simulink model "arducopter"  (R2021a)
settings: Solver=FixedStepAuto  StartTime=0.0  StopTime=sim.param.timeEnd  FixedStep=sim.param.dt  RelTol=1e-3
undefined symbols (not defined in the file or in its folder): DiscIntNeverNeededParam, sim
libraries: simulink x34, slident x4, vrlib x1
(part 4 of 8)

== system arducopter/Attitude Controller/input_euler_angle_roll_pitch_euler_rate_yaw()/update_ang_vel_target_from_att_error() ==
  note: The subsystems either use the square root controller or an easy proportional relation (kp*err) to calculate the target angular velocity
  note: AC_AttitudeControl::update_ang_vel_target_from_att_error()
      | Compute the angular velocity corrections in the body frame from the attitude error.
  attitudeError : Inport
  Calc angular velocity target pitch : Subsystem
  Calc angular velocity target roll : Subsystem
  Calc angular velocity target yaw : Subsystem
  Mux : Mux  Inputs=3
  Selector : Selector  InputPortWidth=3  IndexOptions=Index vector (dialog)  Indices=[1]  OutputSizes=1
  Selector1 : Selector  InputPortWidth=3  IndexOptions=Index vector (dialog)  Indices=[2]  OutputSizes=1
  Selector2 : Selector  InputPortWidth=3  IndexOptions=Index vector (dialog)  Indices=[3]  OutputSizes=1
  angVelBody : Outport
  wires:
  attitudeError/1 -> Selector2/1, Selector/1, Selector1/1
  Mux/1 -> angVelBody/1
  Selector/1 -> Calc angular velocity target roll/1(attitudeErrorRoll)
  Calc angular velocity target roll/1(angVelRoll) -> Mux/1
  Calc angular velocity target yaw/1(angVelYaw) -> Mux/3
  Calc angular velocity target pitch/1(angVelPitch) -> Mux/2
  Selector1/1 -> Calc angular velocity target pitch/1(attitudeErrorPitch)
  Selector2/1 -> Calc angular velocity target yaw/1(attitudeErrorYaw)

== system arducopter/Position Controller/P Position z/Scale Factor Z ==
  note: AP_AHRS::getControlScaleZ()
      | This subsystem calculates a scaling factor for the target of vertical motion quantities based on the EKF type that is being used.
      | Taken from AP_AHRS::getControlScaleZ() in AP_AHRS.cpp. Called in AC_PosControl::update_z_controller().
      | Flying with only DCM lower the gain of the controllers by 4x to cope with high lag.
  ekfType : Inport
  EKF used : Constant  OutDataTypeStr=single
  No EKF : Constant  Value=0.25  OutDataTypeStr=single
  Switch : Switch  Criteria=u2 > Threshold
  scale_z : Outport
  wires:
  ekfType/1 -> Switch/2
  EKF used/1 -> Switch/1
  No EKF/1 -> Switch/3
  Switch/1 -> scale_z/1

== system arducopter/Position Controller/P Position z/Set vertical speed & acceleration limit ==
  note: Calculation of vertical speed and acceleration limits
      | This subsystem corresponds to the function set_correction_speed_accel_z() , in AC_PosControl.cpp,
      | which is called in the ModeLoiter::init() function of mode_loiter.cpp.
      | The intention of this function is to calculate z position error limits, which corresponds to the vertical speed
      | and acceleration limits given by parameters, so that the speed and acceleration limits are still kept after
      | the square root controller was executed without explicitly enforce the limits to the quantities.
  outMin : Inport
  outMax : Inport  Port=2
  DoutMax : Inport  Port=3
  D2OutMax : Inport  Port=4
  kp : Inport  Port=5
  Abs : Abs
  Gain : Gain  Gain=-1
  Inverse Square Root Controller : Subsystem  TreatAsAtomicUnit=on
  Set error limits : MATLAB Function  TreatAsAtomicUnit=on
  errMin : Outport
  errMax : Outport  Port=2
  D1max : Outport  Port=3
  wires:
  Abs/1 -> Gain/1
  Gain/1 -> Set error limits/1(outMin)
  outMax/1 -> Set error limits/2(outMax)
  outMin/1 -> Abs/1
  DoutMax/1 -> Set error limits/3(DoutMax)
  Set error limits/1(errMin) -> errMin/1
  Set error limits/3(D1max) -> D1max/1
  Set error limits/2(errMax) -> errMax/1
  D2OutMax/1 -> Set error limits/4(D2OutMax)
  kp/1 -> Set error limits/5(kp)

== system arducopter/Position Controller/PID Acceleration z/Calc Derivative ==
  e : Inport
  ATC input time constant : Constant  Value=sim.param.dt
  Divide : Product  Inputs=*/
  Sum : Sum  Inputs=|+-
  Unit Delay : UnitDelay  SampleTime=-1  HasFrameUpgradeWarning=on
  derivative : Outport
  wires:
  e/1 -> Sum/1, Unit Delay/1
  Unit Delay/1 -> Sum/2
  Sum/1 -> Divide/1
  ATC input time constant/1 -> Divide/2
  Divide/1 -> derivative/1

== system arducopter/Position Controller/PID Acceleration z/I ==
  note: Integrator, see AC_PID.cpp, line 230
      | Initialization: set_integrator() in AC_PosControl::init_z_controller()
  e : Inport
  limitFlg : Inport  Port=2
  ki : Inport  Port=3
  i_max : Inport  Port=4
  Constant1 : Constant  Value=sim.param.dt
  Data Type Conversion1 : DataTypeConversion  OutDataTypeStr=single
  IC1 : InitialCondition  Value=sim.init.PIDA.I
  Integrator : MATLAB Function  TreatAsAtomicUnit=on
  Unit Delay1 : UnitDelay  InitialCondition=sim.init.PIDA.I  SampleTime=-1  HasFrameUpgradeWarning=on
  integrator : Outport
  wires:
  e/1 -> Integrator/1(error)
  Integrator/1(integrator_out) -> IC1/1
  [integrator_out] -> integrator/1
  Constant1/1 -> Data Type Conversion1/1
  limitFlg/1 -> Integrator/3(limit_flg)
  [integrator_out] -> Unit Delay1/1
  IC1/1 -> [integrator_out]
  Unit Delay1/1 -> Integrator/2(integrator)
  ki/1 -> Integrator/4(ki)
  i_max/1 -> Integrator/5(i_max)
  Data Type Conversion1/1 -> Integrator/6(dt)

== system arducopter/Position Controller/PID Acceleration z/RAT_FLTD ==
  note: Digital Filter:
      | $y_n = (1 - \alpha)y_{n-1} + x \cdot \alpha$
  note: Alpha Calculation:
      | $\alpha = \frac{\mathrm{d}t}{\mathrm{d}t + 2 \pi f_{\mathrm{Cutoff}}$
  note: See AC_PID.cpp, line 144.
  note: See AP_Math.cpp, line 393.
  u : Inport
  cutoff_freq : Inport  Port=2
  ATC input time constant : Constant  Value=sim.param.dt
  Add : Sum
  Calculate Alpha : Product  Inputs=*/
  Compare To Zero : simulink/Logic and Bit Operations/Compare To Zero  relop=<=  OutDataTypeStr=boolean
  Compare To Zero1 : simulink/Logic and Bit Operations/Compare To Zero  relop=<=  OutDataTypeStr=boolean
  Constant2 : Constant  OutDataTypeStr=single
  Constant3 : Constant  OutDataTypeStr=single
  Constant4 : Constant  OutDataTypeStr=single
  Data Type Conversion1 : DataTypeConversion  OutDataTypeStr=single
  Divide : Product  Inputs=*/
  Gain : Gain  Gain=2*pi
  IC : InitialCondition  Value=sim.init.PIDA.DerFilt
  Logical Operator : Logic  Operator=OR  AllPortsSameDT=off  OutDataTypeStr=boolean
  Product : Product
  Product1 : Product
  Subtract1 : Sum  Inputs=+-
  Sum : Sum  Inputs=++|  OutDataTypeStr=single
  Switch : Switch  Criteria=u2 > Threshold
  Unit Delay : UnitDelay  SampleTime=-1  HasFrameUpgradeWarning=on
  y : Outport
  wires:
  Product1/1 -> Sum/2
  Unit Delay/1 -> Product1/2
  Subtract1/1 -> Product1/1
  [alpha] -> Subtract1/2
  Constant2/1 -> Subtract1/1
  [alpha] -> Product/1
  Calculate Alpha/1 -> Switch/3
  Add/1 -> Calculate Alpha/2
  [dt] -> Add/1, Calculate Alpha/1
  Gain/1 -> Divide/2
  cutoff_freq/1 -> [cutoff_freq]
  u/1 -> Product/2
  Divide/1 -> Add/2
  Constant3/1 -> Divide/1
  Product/1 -> Sum/1
  Switch/1 -> [alpha]
  ATC input time constant/1 -> Data Type Conversion1/1
  [cutoff_freq] -> Gain/1
  [dt] -> Compare To Zero/1
  [cutoff_freq] -> Compare To Zero1/1
  Compare To Zero/1 -> Logical Operator/1
  Compare To Zero1/1 -> Logical Operator/2
  Logical Operator/1 -> Switch/2
  Constant4/1 -> Switch/1
  Sum/1 -> IC/1
  IC/1 -> Unit Delay/1, y/1
  Data Type Conversion1/1 -> [dt]

== system arducopter/Position Controller/PID Acceleration z/RAT_FLTE ==
  note: Digital Filter:
      | $y_n = (1 - \alpha)y_{n-1} + x \cdot \alpha$
  note: Alpha Calculation:
      | $\alpha = \frac{\mathrm{d}t}{\mathrm{d}t + 2 \pi f_{\mathrm{Cutoff}}$
  note: See AC_PID.cpp, line 144.
  note: See AP_Math.cpp, line 393.
  u : Inport
  cutoff_freq : Inport  Port=2
  ATC input time constant : Constant  Value=sim.param.dt
  Add : Sum
  Calculate Alpha : Product  Inputs=*/
  Compare To Zero : simulink/Logic and Bit Operations/Compare To Zero  relop=<=  OutDataTypeStr=boolean
  Compare To Zero1 : simulink/Logic and Bit Operations/Compare To Zero  relop=<=  OutDataTypeStr=boolean
  Constant2 : Constant  OutDataTypeStr=single
  Constant3 : Constant  OutDataTypeStr=single
  Constant4 : Constant  OutDataTypeStr=single
  Data Type Conversion1 : DataTypeConversion  OutDataTypeStr=single
  Divide : Product  Inputs=*/
  Gain : Gain  Gain=2*pi
  IC : InitialCondition  Value=sim.init.PIDA.ErrFilt
  Logical Operator : Logic  Operator=OR  AllPortsSameDT=off  OutDataTypeStr=boolean
  Product : Product
  Product1 : Product
  Subtract1 : Sum  Inputs=+-
  Sum : Sum  Inputs=++|  OutDataTypeStr=single
  Switch : Switch  Criteria=u2 > Threshold
  Unit Delay : UnitDelay  SampleTime=-1  HasFrameUpgradeWarning=on
  y : Outport
  wires:
  Product1/1 -> Sum/2
  Unit Delay/1 -> Product1/2
  Subtract1/1 -> Product1/1
  [alpha] -> Subtract1/2
  Constant2/1 -> Subtract1/1
  [alpha] -> Product/1
  Calculate Alpha/1 -> Switch/3
  Add/1 -> Calculate Alpha/2
  [dt] -> Add/1, Calculate Alpha/1
  Gain/1 -> Divide/2
  cutoff_freq/1 -> [cutoff_freq]
  u/1 -> Product/2
  Divide/1 -> Add/2
  Constant3/1 -> Divide/1
  Product/1 -> Sum/1
  Switch/1 -> [alpha]
  ATC input time constant/1 -> Data Type Conversion1/1
  [cutoff_freq] -> Gain/1
  [dt] -> Compare To Zero/1
  [cutoff_freq] -> Compare To Zero1/1
  Compare To Zero/1 -> Logical Operator/1
  Compare To Zero1/1 -> Logical Operator/2
  Logical Operator/1 -> Switch/2
  Constant4/1 -> Switch/1
  Sum/1 -> IC/1
  IC/1 -> Unit Delay/1, y/1
  Data Type Conversion1/1 -> [dt]

== system arducopter/Position Controller/PID Acceleration z/RAT_FLTT ==
  note: See AP_Math.cpp, line 393.
  note: See AC_PID.cpp, line 144.
  note: Alpha Calculation:
      | $\alpha = \frac{\mathrm{d}t}{\mathrm{d}t + 2 \pi f_{\mathrm{Cutoff}}$
  note: Digital Filter:
      | $y_n = (1 - \alpha)y_{n-1} + x \cdot \alpha$
  u : Inport
  cutoff_freq : Inport  Port=2
  ATC input time constant : Constant  Value=sim.param.dt
  Add : Sum
  Calculate Alpha : Product  Inputs=*/
  Compare To Zero : simulink/Logic and Bit Operations/Compare To Zero  relop=<=  OutDataTypeStr=boolean
  Compare To Zero1 : simulink/Logic and Bit Operations/Compare To Zero  relop=<=  OutDataTypeStr=boolean
  Constant2 : Constant  OutDataTypeStr=single
  Constant3 : Constant  OutDataTypeStr=single
  Constant4 : Constant  OutDataTypeStr=single
  Data Type Conversion1 : DataTypeConversion  OutDataTypeStr=single
  Divide : Product  Inputs=*/
  Gain : Gain  Gain=2*pi
  IC : InitialCondition  Value=sim.init.PIDA.TarFilt
  Logical Operator : Logic  Operator=OR  AllPortsSameDT=off  OutDataTypeStr=boolean
  Product : Product
  Product1 : Product
  Subtract1 : Sum  Inputs=+-
  Sum : Sum  Inputs=++|
  Switch : Switch  Criteria=u2 > Threshold
  Unit Delay : UnitDelay  SampleTime=-1  HasFrameUpgradeWarning=on
  y : Outport
  wires:
  Constant4/1 -> Switch/1
  Logical Operator/1 -> Switch/2
  Compare To Zero1/1 -> Logical Operator/2
  Compare To Zero/1 -> Logical Operator/1
  [cutoff_freq] -> Compare To Zero1/1
  [dt] -> Compare To Zero/1
  [cutoff_freq] -> Gain/1
  ATC input time constant/1 -> Data Type Conversion1/1
  Switch/1 -> [alpha]
  Product/1 -> Sum/1
  Constant3/1 -> Divide/1
  Divide/1 -> Add/2
  u/1 -> Product/2
  cutoff_freq/1 -> [cutoff_freq]
  Gain/1 -> Divide/2
  [dt] -> Calculate Alpha/1, Add/1
  Add/1 -> Calculate Alpha/2
  Calculate Alpha/1 -> Switch/3
  [alpha] -> Product/1
  Constant2/1 -> Subtract1/1
  [alpha] -> Subtract1/2
  Subtract1/1 -> Product1/1
  Product1/1 -> Sum/2
  Sum/1 -> IC/1
  Unit Delay/1 -> Product1/2
  IC/1 -> y/1, Unit Delay/1
  Data Type Conversion1/1 -> [dt]

== system arducopter/Position Controller/PID Acceleration z/Slew Limiter ==
  note: Data Store Memory Elements: Global variables of subsystem
  note: Slew Limiter
      |
      | Calculates the slew limit modifiert Dmod for the P and D part of the controller. The calculation of Dmod is taken from SlewLimiter::modifier() in SlewLimiter.cpp.
  p_out : Inport
  sr_max : Inport  Port=2
  sr_tau : Inport  Port=3
  sr_flt_f : Inport  Port=4
  clock : Inport  Port=5
  d_out : Inport  Port=6
  ATC sample time1 : Constant  Value=sim.param.dt
  Calculate Dmod : MATLAB Function  TreatAsAtomicUnit=on
  Constant7 : Constant  Value=sim.param.LOOP_RATE
  Data Store Memory : DataStoreMemory  DataStoreName=pos_event_stored  ReadBeforeWriteMsg=warning  WriteAfterWriteMsg=warning  WriteAfterReadMsg=warning  InitialValue=false  ShowAdditionalParam=off  OutDataTypeStr=boolean
  Data Store Memory1 : DataStoreMemory  DataStoreName=neg_event_stored  ReadBeforeWriteMsg=warning  WriteAfterWriteMsg=warning  WriteAfterReadMsg=warning  InitialValue=false  ShowAdditionalParam=off  OutDataTypeStr=boolean
  Data Store Memory10 : DataStoreMemory  DataStoreName=modifier_slew_rate  ReadBeforeWriteMsg=warning  WriteAfterWriteMsg=warning  WriteAfterReadMsg=warning  InitialValue=sim.init.PIDA.SROut  ShowAdditionalParam=off  OutDataTypeStr=single
  Data Store Memory11 : DataStoreMemory  DataStoreName=output_slew_rate  ReadBeforeWriteMsg=warning  WriteAfterWriteMsg=warning  WriteAfterReadMsg=warning  InitialValue=sim.init.PIDA.SROut  ShowAdditionalParam=off  OutDataTypeStr=single
  Data Store Memory2 : DataStoreMemory  DataStoreName=pos_event_idx  ReadBeforeWriteMsg=warning  WriteAfterWriteMsg=warning  WriteAfterReadMsg=warning  InitialValue=1  ShowAdditionalParam=off  OutDataTypeStr=int8
  Data Store Memory3 : DataStoreMemory  DataStoreName=neg_event_idx  ReadBeforeWriteMsg=warning  WriteAfterWriteMsg=warning  WriteAfterReadMsg=warning  InitialValue=1  ShowAdditionalParam=off  OutDataTypeStr=int8
  Data Store Memory4 : DataStoreMemory  DataStoreName=pos_event_ms  ReadBeforeWriteMsg=warning  WriteAfterWriteMsg=warning  WriteAfterReadMsg=warning  InitialValue=[0 0]  ShowAdditionalParam=off  OutDataTypeStr=uint32  Dimensions=2
  Data Store Memory5 : DataStoreMemory  DataStoreName=neg_event_ms  ReadBeforeWriteMsg=warning  WriteAfterWriteMsg=warning  WriteAfterReadMsg=warning  InitialValue=[0 0]  ShowAdditionalParam=off  OutDataTypeStr=uint32  Dimensions=2
  Data Store Memory6 : DataStoreMemory  DataStoreName=max_pos_slew_rate  ReadBeforeWriteMsg=warning  WriteAfterWriteMsg=warning  WriteAfterReadMsg=warning  ShowAdditionalParam=off  OutDataTypeStr=single
  Data Store Memory7 : DataStoreMemory  DataStoreName=max_pos_slew_event_ms  ReadBeforeWriteMsg=warning  WriteAfterWriteMsg=warning  WriteAfterReadMsg=warning  ShowAdditionalParam=off  OutDataTypeStr=uint32
  Data Store Memory8 : DataStoreMemory  DataStoreName=max_neg_slew_rate  ReadBeforeWriteMsg=warning  WriteAfterWriteMsg=warning  WriteAfterReadMsg=warning  ShowAdditionalParam=off  OutDataTypeStr=single
  Data Store Memory9 : DataStoreMemory  DataStoreName=max_neg_slew_event_ms  ReadBeforeWriteMsg=warning  WriteAfterWriteMsg=warning  WriteAfterReadMsg=warning  ShowAdditionalParam=off  OutDataTypeStr=uint32
  Data Store Read : DataStoreRead  DataStoreName=modifier_slew_rate  DataStoreElements=modifier_slew_rate  IndexOptions=Index vector (dialog)  Indices=1  OutputSizes=1
  Data Store Read1 : DataStoreRead  DataStoreName=output_slew_rate  DataStoreElements=output_slew_rate  IndexOptions=Index vector (dialog)  Indices=1  OutputSizes=1
  Data Type Conversion1 : DataTypeConversion  OutDataTypeStr=single
  IC : InitialCondition  Value=2*sim.init.PIDA.SROut
  Lowpass Filter : MATLAB Function  TreatAsAtomicUnit=on
  Subsystem : Subsystem
  Terminator : Terminator
  Terminator1 : Terminator
  Unit Delay1 : UnitDelay  SampleTime=-1  HasFrameUpgradeWarning=on
  Dmod : Outport
  wires:
  Constant7/1 -> Lowpass Filter/3(loop_rate)
  sr_flt_f/1 -> Lowpass Filter/2(cutoff_freq)
  Lowpass Filter/1(out) -> IC/1  "zAccSrFilt"
  Unit Delay1/1 -> Lowpass Filter/4(out_last)
  Calculate Dmod/1(Dmod) -> Dmod/1  "zAccDmod"
  sr_max/1 -> Calculate Dmod/2(sr_max)
  sr_tau/1 -> Calculate Dmod/3(sr_tau)
  ATC sample time1/1 -> Data Type Conversion1/1
  Data Store Read/1 -> Terminator/1  "zAccSrMod"
  Data Store Read1/1 -> Terminator1/1  "zAccSrOut"
  p_out/1 -> Subsystem/1(p_out)
  d_out/1 -> Subsystem/2(d_out)
  Subsystem/1(sr_raw) -> Lowpass Filter/1(in)  "zAccSrRaw"
  Data Type Conversion1/1 -> Calculate Dmod/4(dt)
  IC/1 -> Unit Delay1/1, Calculate Dmod/1(slew_rate)
  clock/1 -> Calculate Dmod/5(time)

== system arducopter/Position Controller/PID Acceleration z/i_max check ==
  note: Ensure imax is always large enough to overpower hover throttle
      | Check for sufficient high imax is taken from AC_PosControl.cpp, line 984-986.
  thrHover : Inport
  i_max_ : Inport  Port=2
  Gain : Gain  Gain=1000
  Relational Operator : RelationalOperator  Operator=>  OutDataTypeStr=boolean  RndMeth=Simplest
  Switch : Switch  Criteria=u2 > Threshold
  i_max : Outport
  wires:
  thrHover/1 -> Gain/1
  Gain/1 -> Switch/1, Relational Operator/1
  i_max_/1 -> Switch/3, Relational Operator/2
  Relational Operator/1 -> Switch/2
  Switch/1 -> i_max/1

== system arducopter/Position Controller/PID Velocity z/Calc Derivative ==
  e : Inport
  ATC input time constant : Constant  Value=sim.param.dt
  Divide : Product  Inputs=*/
  Sum : Sum  Inputs=|+-
  Unit Delay : UnitDelay  SampleTime=-1  HasFrameUpgradeWarning=on
  derivative : Outport
  wires:
  e/1 -> Sum/1, Unit Delay/1
  Unit Delay/1 -> Sum/2
  Sum/1 -> Divide/1
  ATC input time constant/1 -> Divide/2
  Divide/1 -> derivative/1

== system arducopter/Position Controller/PID Velocity z/I ==
  note: Integrator, see AC_PID_Basic::update_i()
      | Initialization: integrator=0 (see AC_PosControl::init_z())
  e : Inport
  limitNeg : Inport  Port=2
  limitPos : Inport  Port=3
  ki : Inport  Port=4
  i_max : Inport  Port=5
  Constant1 : Constant  Value=sim.param.dt
  Data Type Conversion1 : DataTypeConversion  OutDataTypeStr=single
  IC1 : InitialCondition  Value=0
  Integrator : MATLAB Function  TreatAsAtomicUnit=on
  Unit Delay1 : UnitDelay  InitialCondition=single(0)  SampleTime=-1  HasFrameUpgradeWarning=on
  integrator : Outport
  wires:
  e/1 -> Integrator/1(error)
  Integrator/1(integrator_out) -> IC1/1
  [integrator_out] -> integrator/1
  Constant1/1 -> Data Type Conversion1/1
  limitNeg/1 -> Integrator/3(limitNeg)
  [integrator_out] -> Unit Delay1/1
  IC1/1 -> [integrator_out]
  Unit Delay1/1 -> Integrator/2(integrator)
  ki/1 -> Integrator/5(ki)
  i_max/1 -> Integrator/6(i_max)
  Data Type Conversion1/1 -> Integrator/7(dt)
  limitPos/1 -> Integrator/4(limitPos)

== system arducopter/Position Controller/PID Velocity z/RAT_FLTD ==
  note: Digital Filter:
      | $y_n = (1 - \alpha)y_{n-1} + x \cdot \alpha$
  note: Alpha Calculation:
      | $\alpha = \frac{\mathrm{d}t}{\mathrm{d}t + 2 \pi f_{\mathrm{Cutoff}}$
  note: See AC_PID.cpp, update_all()
  note: See AP_Math.cpp, calc_lowpass_alpha_dt()
  u : Inport
  cutoff_freq : Inport  Port=2
  ATC input time constant : Constant  Value=sim.param.dt
  Add : Sum
  Calculate Alpha : Product  Inputs=*/
  Compare To Zero : simulink/Logic and Bit Operations/Compare To Zero  relop=<=  OutDataTypeStr=boolean
  Compare To Zero1 : simulink/Logic and Bit Operations/Compare To Zero  relop=<=  OutDataTypeStr=boolean
  Constant2 : Constant  OutDataTypeStr=single
  Constant3 : Constant  OutDataTypeStr=single
  Constant4 : Constant  OutDataTypeStr=single
  Data Type Conversion1 : DataTypeConversion  OutDataTypeStr=single
  Divide : Product  Inputs=*/
  Gain : Gain  Gain=2*pi
  IC : InitialCondition  Value=0
  Logical Operator : Logic  Operator=OR  AllPortsSameDT=off  OutDataTypeStr=boolean
  Product : Product
  Product1 : Product
  Subtract1 : Sum  Inputs=+-
  Sum : Sum  Inputs=++|  OutDataTypeStr=single
  Switch : Switch  Criteria=u2 > Threshold
  Unit Delay : UnitDelay  SampleTime=-1  HasFrameUpgradeWarning=on
  y : Outport
  wires:
  Product1/1 -> Sum/2
  Unit Delay/1 -> Product1/2
  Subtract1/1 -> Product1/1
  [alpha] -> Subtract1/2
  Constant2/1 -> Subtract1/1
  [alpha] -> Product/1
  Calculate Alpha/1 -> Switch/3
  Add/1 -> Calculate Alpha/2
  [dt] -> Add/1, Calculate Alpha/1
  Gain/1 -> Divide/2
  cutoff_freq/1 -> [cutoff_freq]
  u/1 -> Product/2
  Divide/1 -> Add/2
  Constant3/1 -> Divide/1
  Product/1 -> Sum/1
  Switch/1 -> [alpha]
  ATC input time constant/1 -> Data Type Conversion1/1
  [cutoff_freq] -> Gain/1
  [dt] -> Compare To Zero/1
  [cutoff_freq] -> Compare To Zero1/1
  Compare To Zero/1 -> Logical Operator/1
  Compare To Zero1/1 -> Logical Operator/2
  Logical Operator/1 -> Switch/2
  Constant4/1 -> Switch/1
  Sum/1 -> IC/1
  IC/1 -> Unit Delay/1, y/1
  Data Type Conversion1/1 -> [dt]

== system arducopter/Position Controller/PID Velocity z/RAT_FLTE ==
  note: Digital Filter:
      | $y_n = (1 - \alpha)y_{n-1} + x \cdot \alpha$
  note: Alpha Calculation:
      | $\alpha = \frac{\mathrm{d}t}{\mathrm{d}t + 2 \pi f_{\mathrm{Cutoff}}$
  note: See AC_PID.cpp, update_all()
  note: See AP_Math.cpp, calc_lowpass_alpha_dt()
  u : Inport
  cutoff_freq : Inport  Port=2
  ATC input time constant : Constant  Value=sim.param.dt
  Add : Sum
  Calculate Alpha : Product  Inputs=*/
  Compare To Zero : simulink/Logic and Bit Operations/Compare To Zero  relop=<=  OutDataTypeStr=boolean
  Compare To Zero1 : simulink/Logic and Bit Operations/Compare To Zero  relop=<=  OutDataTypeStr=boolean
  Constant2 : Constant  OutDataTypeStr=single
  Constant3 : Constant  OutDataTypeStr=single
  Constant4 : Constant  OutDataTypeStr=single
  Data Type Conversion1 : DataTypeConversion  OutDataTypeStr=single
  Divide : Product  Inputs=*/
  Gain : Gain  Gain=2*pi
  IC : InitialCondition  Value=0
  Logical Operator : Logic  Operator=OR  AllPortsSameDT=off  OutDataTypeStr=boolean
  Product : Product
  Product1 : Product
  Subtract1 : Sum  Inputs=+-
  Sum : Sum  Inputs=++|  OutDataTypeStr=single
  Switch : Switch  Criteria=u2 > Threshold
  Unit Delay : UnitDelay  SampleTime=-1  HasFrameUpgradeWarning=on
  y : Outport
  wires:
  Product1/1 -> Sum/2
  Unit Delay/1 -> Product1/2
  Subtract1/1 -> Product1/1
  [alpha] -> Subtract1/2
  Constant2/1 -> Subtract1/1
  [alpha] -> Product/1
  Calculate Alpha/1 -> Switch/3
  Add/1 -> Calculate Alpha/2
  [dt] -> Add/1, Calculate Alpha/1
  Gain/1 -> Divide/2
  cutoff_freq/1 -> [cutoff_freq]
  u/1 -> Product/2
  Divide/1 -> Add/2
  Constant3/1 -> Divide/1
  Product/1 -> Sum/1
  Switch/1 -> [alpha]
  ATC input time constant/1 -> Data Type Conversion1/1
  [cutoff_freq] -> Gain/1
  [dt] -> Compare To Zero/1
  [cutoff_freq] -> Compare To Zero1/1
  Compare To Zero/1 -> Logical Operator/1
  Compare To Zero1/1 -> Logical Operator/2
  Logical Operator/1 -> Switch/2
  Constant4/1 -> Switch/1
  Sum/1 -> IC/1
  IC/1 -> Unit Delay/1, y/1
  Data Type Conversion1/1 -> [dt]

== system arducopter/Position Controller/PID Velocity z/Scale Factor Z ==
  note: AP_AHRS::getControlScaleZ()
      | This subsystem calculates a scaling factor for the target of vertical motion quantities based on the EKF type that is being used.
      | Taken from AP_AHRS::getControlScaleZ() in AP_AHRS.cpp. Called in AC_PosControl::update_z_controller().
      | Flying with only DCM lower the gain of the controllers by 4x to cope with high lag.
  ekfType : Inport
  EKF used : Constant  OutDataTypeStr=single
  No EKF : Constant  Value=0.25  OutDataTypeStr=single
  Switch : Switch  Criteria=u2 > Threshold
  scale_z : Outport
  wires:
  ekfType/1 -> Switch/2
  EKF used/1 -> Switch/1
  No EKF/1 -> Switch/3
  Switch/1 -> scale_z/1

== system arducopter/Position Controller/calc des climb rate/contrain climb rate ==
  note: Based on get_pilot_speed_dn()
      | Use maximum up-speed if down-speed limit is 0
  in : Inport
  Abs : Abs
  Abs1 : Abs
  Constant1 : Constant  Value=sim.param.PSCD.VEL_MAX_DN
  Constant2 : Constant  Value=sim.param.PSCD.VEL_MAX_UP
  Constant3 : Constant  Value=sim.param.PSCD.VEL_MAX_UP
  Gain : Gain  Gain=-1
  Saturation Dynamic : simulink/Discontinuities/Saturation Dynamic  OutMin=[]  OutMax=[]  OutDataTypeStr=Inherit: Same as second input  OutDataType=fixdt(1, 16)  OutScaling=2^-10  DoSatur=off
  Switch : Switch  Criteria=u2 > Threshold
  out : Outport
  wires:
  Constant1/1 -> Abs/1, Switch/2
  Constant2/1 -> Abs1/1
  Abs/1 -> Switch/1
  Abs1/1 -> Switch/3
  Saturation Dynamic/1 -> out/1
  Switch/1 -> Gain/1
  Gain/1 -> Saturation Dynamic/3
  in/1 -> Saturation Dynamic/2
  Constant3/1 -> Saturation Dynamic/1

== system arducopter/Position Controller/set_pos_target_z_from_climb_rate()/input_vel_accel_z ==
  note: input_vel_accel_z()
      | This subsystem takes the current target position (posTarIn) and desired velocity and acceleration (velDesTar and accDesTar).
      | First, it updates the target position and desired velocity based on the current desired acceleration (accDesIn) (1).
      | Secondly, it calculates the required jerk limited adjustment to the acceleration for the next time dt (accDes) to reach the desired velocity and acceleration targets (velDesTar and accDesTar) (2).
  note: (2) shape_vel_accel()
      | Adjustment of the desired acceleration to follow a jerk limited kinematic path to vel and acc
  note: (1) update_pos_vel_accel()
      | Adjust desired position and velocity based on desired acceleration
  note: Calculate overspeed gain to calculate increased max accel and jerk if over speed
  velDesTar : Inport
  accDesTar : Inport  Port=2
  limitVectorZ : Inport  Port=3
  velMaxUp : Inport  Port=4
  velMaxDn : Inport  Port=5
  accMaxZ : Inport  Port=6
  jerkMax : Inport  Port=7
  posTarIn : Inport  Port=8
  posErr : Inport  Port=9
  velErr : Inport  Port=10
  velDesIn : Inport  Port=11
  accDesIn : Inport  Port=12
  Constant : Constant  Value=sim.param.PSCD.OVERSPEED_GAIN_Z
  Constant1 : Constant  OutDataTypeStr=boolean
  Constant2 : Constant  Value=sim.param.dt  OutDataTypeStr=single
  MATLAB Function : MATLAB Function  TreatAsAtomicUnit=on
  Product : Product
  Product1 : Product
  calc accMin : Subsystem
  shape_vel_accel : Subsystem
  update_pos_vel_accel : Subsystem
  posTar : Outport
  velDes : Outport  Port=2
  accDes : Outport  Port=3
  wires:
  velMaxUp/1 -> MATLAB Function/1(velMaxUp)
  accMaxZ/1 -> Product/2
  velDesIn/1 -> [velDesIn]
  velMaxDn/1 -> MATLAB Function/2(velMaxDn)
  Constant/1 -> MATLAB Function/4(overspeedGainDefault)
  [velDesIn] -> MATLAB Function/3(velDes)
  posTarIn/1 -> update_pos_vel_accel/1(posTarIn)
  [velDesIn] -> update_pos_vel_accel/2(velDesIn)
  accDesIn/1 -> [accDesIn]
  limitVectorZ/1 -> update_pos_vel_accel/4(limitVectorZ)
  update_pos_vel_accel/2(velDes) -> [velDes]
  accDesTar/1 -> shape_vel_accel/2(acc)
  velDesTar/1 -> shape_vel_accel/1(vel)
  [accDesIn] -> update_pos_vel_accel/3(accDesIn)
  [accDesIn] -> shape_vel_accel/4(accDes)
  [accMax] -> calc accMin/1(accMax), shape_vel_accel/6(accMax)
  calc accMin/1(accMin) -> shape_vel_accel/5(accMin)
  Constant2/1 -> shape_vel_accel/8(dt)
  Constant1/1 -> shape_vel_accel/9(limitTotalAccel)
  update_pos_vel_accel/1(posTar) -> posTar/1
  [velDes] -> shape_vel_accel/3(velDes)
  [velDes] -> velDes/1
  shape_vel_accel/1(accDesShaped) -> accDes/1
  MATLAB Function/1(overspeedGain) -> Product1/1, Product/1
  Product/1 -> [accMax]
  jerkMax/1 -> Product1/2
  Product1/1 -> [jerkMax]
  [jerkMax] -> shape_vel_accel/7(jerkMax)
  posErr/1 -> update_pos_vel_accel/5(posErr)
  velErr/1 -> update_pos_vel_accel/6(velErr)

== system arducopter/Rate Controller/PID Pitch Rate/Calc Derivative ==
  e : Inport
  ATC input time constant : Constant  Value=sim.param.dt
  Data Type Conversion1 : DataTypeConversion  OutDataTypeStr=single
  Divide : Product  Inputs=*/
  Sum : Sum  Inputs=|+-
  Unit Delay : UnitDelay  SampleTime=-1  HasFrameUpgradeWarning=on
  derivative : Outport
  wires:
  Divide/1 -> derivative/1
  ATC input time constant/1 -> Data Type Conversion1/1
  Sum/1 -> Divide/1
  Unit Delay/1 -> Sum/2
  e/1 -> Unit Delay/1, Sum/1
  Data Type Conversion1/1 -> Divide/2

== system arducopter/Rate Controller/PID Pitch Rate/I ==
  note: Integrator, see AC_PID::update_i()
  e : Inport
  limit_flg : Inport  Port=2
  ki : Inport  Port=3
  i_max : Inport  Port=4
  Constant1 : Constant  Value=sim.param.dt
  Data Type Conversion1 : DataTypeConversion  OutDataTypeStr=single
  IC1 : InitialCondition  Value=sim.init.PIDP.I
  Integrator : MATLAB Function  TreatAsAtomicUnit=on
  Unit Delay1 : UnitDelay  InitialCondition=single(0)  SampleTime=-1  HasFrameUpgradeWarning=on
  integrator : Outport
  wires:
  i_max/1 -> Integrator/5(i_max)
  ki/1 -> Integrator/4(ki)
  Unit Delay1/1 -> Integrator/2(integrator)
  IC1/1 -> [integrator_out]
  [integrator_out] -> Unit Delay1/1
  limit_flg/1 -> Integrator/3(limit_flg)
  Constant1/1 -> Data Type Conversion1/1
  [integrator_out] -> integrator/1
  Integrator/1(integrator_out) -> IC1/1
  e/1 -> Integrator/1(error)
  Data Type Conversion1/1 -> Integrator/6(dt)

== system arducopter/Rate Controller/PID Pitch Rate/RAT_FLTD ==
  note: See AP_Math.cpp, calc_lowpass_alpha_dt()
  note: See AC_PID.cpp, update_all()
  note: Alpha Calculation:
      | $\alpha = \frac{\mathrm{d}t}{\mathrm{d}t + 2 \pi f_{\mathrm{Cutoff}}$
  note: Digital Filter:
      | $y_n = (1 - \alpha)y_{n-1} + x \cdot \alpha$
  u : Inport
  cutoff_freq : Inport  Port=2
  ATC input time constant : Constant  Value=sim.param.dt
  Add : Sum
  Calculate Alpha : Product  Inputs=*/
  Compare To Zero : simulink/Logic and Bit Operations/Compare To Zero  relop=<=  OutDataTypeStr=boolean
  Compare To Zero1 : simulink/Logic and Bit Operations/Compare To Zero  relop=<=  OutDataTypeStr=boolean
  Constant2 : Constant  OutDataTypeStr=single
  Constant3 : Constant  OutDataTypeStr=single
  Constant4 : Constant  OutDataTypeStr=single
  Data Type Conversion1 : DataTypeConversion  OutDataTypeStr=single
  Divide : Product  Inputs=*/
  Gain : Gain  Gain=2*pi
  IC : InitialCondition  Value=sim.init.PIDP.DerFilt
  Logical Operator : Logic  Operator=OR  AllPortsSameDT=off  OutDataTypeStr=boolean
  Product : Product
  Product1 : Product
  Subtract1 : Sum  Inputs=+-
  Sum : Sum  Inputs=++|
  Switch : Switch  Criteria=u2 > Threshold
  Unit Delay : UnitDelay  SampleTime=-1  HasFrameUpgradeWarning=on
  y : Outport
  wires:
  IC/1 -> y/1, Unit Delay/1
  Sum/1 -> IC/1
  Constant4/1 -> Switch/1
  Logical Operator/1 -> Switch/2
  Compare To Zero1/1 -> Logical Operator/2
  Compare To Zero/1 -> Logical Operator/1
  [cutoff_freq] -> Compare To Zero1/1
  [dt] -> Compare To Zero/1
  [cutoff_freq] -> Gain/1
  ATC input time constant/1 -> Data Type Conversion1/1
  Switch/1 -> [alpha]
  Product/1 -> Sum/1
  Constant3/1 -> Divide/1
  Divide/1 -> Add/2
  u/1 -> Product/2
  cutoff_freq/1 -> [cutoff_freq]
  Gain/1 -> Divide/2
  [dt] -> Calculate Alpha/1, Add/1
  Add/1 -> Calculate Alpha/2
  Calculate Alpha/1 -> Switch/3
  [alpha] -> Product/1
  Constant2/1 -> Subtract1/1
  [alpha] -> Subtract1/2
  Subtract1/1 -> Product1/1
  Unit Delay/1 -> Product1/2
  Product1/1 -> Sum/2
  Data Type Conversion1/1 -> [dt]

== system arducopter/Rate Controller/PID Pitch Rate/RAT_FLTE ==
  note: See AP_Math.cpp, calc_lowpass_alpha_dt()
  note: See AC_PID.cpp, update_all()
  note: Alpha Calculation:
      | $\alpha = \frac{\mathrm{d}t}{\mathrm{d}t + 2 \pi f_{\mathrm{Cutoff}}$
  note: Digital Filter:
      | $y_n = (1 - \alpha)y_{n-1} + x \cdot \alpha$
  u : Inport
  cutoff_freq : Inport  Port=2
  ATC input time constant : Constant  Value=sim.param.dt
  Add : Sum
  Calculate Alpha : Product  Inputs=*/
  Compare To Zero : simulink/Logic and Bit Operations/Compare To Zero  relop=<=  OutDataTypeStr=boolean
  Compare To Zero1 : simulink/Logic and Bit Operations/Compare To Zero  relop=<=  OutDataTypeStr=boolean
  Constant2 : Constant  OutDataTypeStr=single
  Constant3 : Constant  OutDataTypeStr=single
  Constant4 : Constant  OutDataTypeStr=single
  Data Type Conversion1 : DataTypeConversion  OutDataTypeStr=single
  Divide : Product  Inputs=*/
  Gain : Gain  Gain=2*pi
  IC : InitialCondition  Value=sim.init.PIDP.ErrFilt
  Logical Operator : Logic  Operator=OR  AllPortsSameDT=off  OutDataTypeStr=boolean
  Product : Product
  Product1 : Product
  Subtract1 : Sum  Inputs=+-
  Sum : Sum  Inputs=++|  OutDataTypeStr=single
  Switch : Switch  Criteria=u2 > Threshold
  Unit Delay : UnitDelay  SampleTime=-1  HasFrameUpgradeWarning=on
  y : Outport
  wires:
  IC/1 -> y/1, Unit Delay/1
  Sum/1 -> IC/1
  Constant4/1 -> Switch/1
  Logical Operator/1 -> Switch/2
  Compare To Zero1/1 -> Logical Operator/2
  Compare To Zero/1 -> Logical Operator/1
  [cutoff_freq] -> Compare To Zero1/1
  [dt] -> Compare To Zero/1
  [cutoff_freq] -> Gain/1
  ATC input time constant/1 -> Data Type Conversion1/1
  Switch/1 -> [alpha]
  Product/1 -> Sum/1
  Constant3/1 -> Divide/1
  Divide/1 -> Add/2
  u/1 -> Product/2
  cutoff_freq/1 -> [cutoff_freq]
  Gain/1 -> Divide/2
  [dt] -> Calculate Alpha/1, Add/1
  Add/1 -> Calculate Alpha/2
  Calculate Alpha/1 -> Switch/3
  [alpha] -> Product/1
  Constant2/1 -> Subtract1/1
  [alpha] -> Subtract1/2
  Subtract1/1 -> Product1/1
  Unit Delay/1 -> Product1/2
  Product1/1 -> Sum/2
  Data Type Conversion1/1 -> [dt]

== system arducopter/Rate Controller/PID Pitch Rate/RAT_FLTT ==
  note: Digital Filter:
      | $y_n = (1 - \alpha)y_{n-1} + x \cdot \alpha$
  note: Alpha Calculation:
      | $\alpha = \frac{\mathrm{d}t}{\mathrm{d}t + 2 \pi f_{\mathrm{Cutoff}}$
  note: See AC_PID.cpp, update_all()
  note: See AP_Math.cpp, calc_lowpass_alpha_dt()
  u : Inport
  cutoff_freq : Inport  Port=2
  ATC input time constant : Constant  Value=sim.param.dt
  Add : Sum
  Calculate Alpha : Product  Inputs=*/
  Compare To Zero : simulink/Logic and Bit Operations/Compare To Zero  relop=<=  OutDataTypeStr=boolean
  Compare To Zero1 : simulink/Logic and Bit Operations/Compare To Zero  relop=<=  OutDataTypeStr=boolean
  Constant2 : Constant  OutDataTypeStr=single
  Constant3 : Constant  OutDataTypeStr=single
  Constant4 : Constant  OutDataTypeStr=single
  Data Type Conversion1 : DataTypeConversion  OutDataTypeStr=single
  Divide : Product  Inputs=*/
  Gain : Gain  Gain=2*pi
  IC : InitialCondition  Value=sim.init.PIDP.TarFilt
  Logical Operator : Logic  Operator=OR  AllPortsSameDT=off  OutDataTypeStr=boolean
  Product : Product
  Product1 : Product
  Subtract1 : Sum  Inputs=+-
  Sum : Sum  Inputs=++|
  Switch : Switch  Criteria=u2 > Threshold
  Unit Delay : UnitDelay  SampleTime=-1  HasFrameUpgradeWarning=on
  y : Outport
  wires:
  IC/1 -> Unit Delay/1, y/1
  Unit Delay/1 -> Product1/2
  Sum/1 -> IC/1
  Product1/1 -> Sum/2
  Subtract1/1 -> Product1/1
  [alpha] -> Subtract1/2
  Constant2/1 -> Subtract1/1
  [alpha] -> Product/1
  Calculate Alpha/1 -> Switch/3
  Add/1 -> Calculate Alpha/2
  [dt] -> Add/1, Calculate Alpha/1
  Gain/1 -> Divide/2
  cutoff_freq/1 -> [cutoff_freq]
  u/1 -> Product/2
  Divide/1 -> Add/2
  Constant3/1 -> Divide/1
  Product/1 -> Sum/1
  Switch/1 -> [alpha]
  ATC input time constant/1 -> Data Type Conversion1/1
  [cutoff_freq] -> Gain/1
  [dt] -> Compare To Zero/1
  [cutoff_freq] -> Compare To Zero1/1
  Compare To Zero/1 -> Logical Operator/1
  Compare To Zero1/1 -> Logical Operator/2
  Logical Operator/1 -> Switch/2
  Constant4/1 -> Switch/1
  Data Type Conversion1/1 -> [dt]

== system arducopter/Rate Controller/PID Pitch Rate/Slew Limiter ==
  note: Data Store Memory Elements: Global variables of subsystem
  note: Slew Limiter
      |
      | Calculates the slew limit modifiert Dmod for the P and D part of the controller. The calculation of Dmod is taken from SlewLimiter::modifier() in SlewLimiter.cpp.
  p_out : Inport
  sr_max : Inport  Port=2
  sr_tau : Inport  Port=3
  sr_flt_f : Inport  Port=4
  clock : Inport  Port=5
  d_out : Inport  Port=6
  ATC sample time1 : Constant  Value=sim.param.dt
  Calculate Dmod1 : MATLAB Function  TreatAsAtomicUnit=on  SystemSampleTime=0.0025
  Constant7 : Constant  Value=sim.param.LOOP_RATE
  Data Store Memory : DataStoreMemory  DataStoreName=pos_event_stored  ReadBeforeWriteMsg=warning  WriteAfterWriteMsg=warning  WriteAfterReadMsg=warning  InitialValue=false  ShowAdditionalParam=off  OutDataTypeStr=boolean
  Data Store Memory1 : DataStoreMemory  DataStoreName=neg_event_stored  ReadBeforeWriteMsg=warning  WriteAfterWriteMsg=warning  WriteAfterReadMsg=warning  InitialValue=false  ShowAdditionalParam=off  OutDataTypeStr=boolean
  Data Store Memory10 : DataStoreMemory  DataStoreName=modifier_slew_rate  ReadBeforeWriteMsg=warning  WriteAfterWriteMsg=warning  WriteAfterReadMsg=warning  InitialValue=sim.init.PIDP.SrOut  ShowAdditionalParam=off  OutDataTypeStr=single
  Data Store Memory11 : DataStoreMemory  DataStoreName=output_slew_rate  ReadBeforeWriteMsg=warning  WriteAfterWriteMsg=warning  WriteAfterReadMsg=warning  InitialValue=sim.init.PIDP.SrOut  ShowAdditionalParam=off  OutDataTypeStr=single
  Data Store Memory2 : DataStoreMemory  DataStoreName=pos_event_idx  ReadBeforeWriteMsg=warning  WriteAfterWriteMsg=warning  WriteAfterReadMsg=warning  InitialValue=1  ShowAdditionalParam=off  OutDataTypeStr=int8
  Data Store Memory3 : DataStoreMemory  DataStoreName=neg_event_idx  ReadBeforeWriteMsg=warning  WriteAfterWriteMsg=warning  WriteAfterReadMsg=warning  InitialValue=1  ShowAdditionalParam=off  OutDataTypeStr=int8
  Data Store Memory4 : DataStoreMemory  DataStoreName=pos_event_ms  ReadBeforeWriteMsg=warning  WriteAfterWriteMsg=warning  WriteAfterReadMsg=warning  InitialValue=[0 0]  ShowAdditionalParam=off  OutDataTypeStr=uint32  Dimensions=2
  Data Store Memory5 : DataStoreMemory  DataStoreName=neg_event_ms  ReadBeforeWriteMsg=warning  WriteAfterWriteMsg=warning  WriteAfterReadMsg=warning  InitialValue=[0 0]  ShowAdditionalParam=off  OutDataTypeStr=uint32  Dimensions=2
  Data Store Memory6 : DataStoreMemory  DataStoreName=max_pos_slew_rate  ReadBeforeWriteMsg=warning  WriteAfterWriteMsg=warning  WriteAfterReadMsg=warning  ShowAdditionalParam=off  OutDataTypeStr=single
  Data Store Memory7 : DataStoreMemory  DataStoreName=max_pos_slew_event_ms  ReadBeforeWriteMsg=warning  WriteAfterWriteMsg=warning  WriteAfterReadMsg=warning  ShowAdditionalParam=off  OutDataTypeStr=uint32
  Data Store Memory8 : DataStoreMemory  DataStoreName=max_neg_slew_rate  ReadBeforeWriteMsg=warning  WriteAfterWriteMsg=warning  WriteAfterReadMsg=warning  ShowAdditionalParam=off  OutDataTypeStr=single
  Data Store Memory9 : DataStoreMemory  DataStoreName=max_neg_slew_event_ms  ReadBeforeWriteMsg=warning  WriteAfterWriteMsg=warning  WriteAfterReadMsg=warning  ShowAdditionalParam=off  OutDataTypeStr=uint32
  Data Store Read : DataStoreRead  DataStoreName=modifier_slew_rate  DataStoreElements=modifier_slew_rate  IndexOptions=Index vector (dialog)  Indices=1  OutputSizes=1
  Data Store Read1 : DataStoreRead  DataStoreName=output_slew_rate  DataStoreElements=output_slew_rate  IndexOptions=Index vector (dialog)  Indices=1  OutputSizes=1
  Data Type Conversion1 : DataTypeConversion  OutDataTypeStr=single
  IC : InitialCondition  Value=2*sim.init.PIDP.SrOut
  Lowpass Filter1 : MATLAB Function  TreatAsAtomicUnit=on
  Subsystem : Subsystem
  Terminator : Terminator
  Terminator1 : Terminator
  Unit Delay1 : UnitDelay  SampleTime=-1  HasFrameUpgradeWarning=on
  Dmod : Outport
  wires:
  Constant7/1 -> Lowpass Filter1/3(loop_rate)
  sr_flt_f/1 -> Lowpass Filter1/2(cutoff_freq)
  Lowpass Filter1/1(out) -> IC/1  "pitchRateSrFilt"
  Unit Delay1/1 -> Lowpass Filter1/4(out_last)
  Calculate Dmod1/1(Dmod) -> Dmod/1  "pitchRateDmod"
  sr_max/1 -> Calculate Dmod1/2(sr_max)
  sr_tau/1 -> Calculate Dmod1/3(sr_tau)
  ATC sample time1/1 -> Data Type Conversion1/1
  Data Store Read/1 -> Terminator/1  "pitchRateSrMod"
  Data Store Read1/1 -> Terminator1/1  "pitchRateSrOut"
  p_out/1 -> Subsystem/1(p_out)
  d_out/1 -> Subsystem/2(d_out)
  Subsystem/1(sr_raw) -> Lowpass Filter1/1(in)  "pitchRateSrRaw"
  Data Type Conversion1/1 -> Calculate Dmod1/4(dt)
  IC/1 -> Calculate Dmod1/1(slew_rate), Unit Delay1/1
  clock/1 -> Calculate Dmod1/5(time)

== system arducopter/Rate Controller/PID Roll Rate/Calc Derivative ==
  e : Inport
  ATC input time constant : Constant  Value=sim.param.dt
  Data Type Conversion : DataTypeConversion  OutDataTypeStr=single
  Divide : Product  Inputs=*/
  Sum : Sum  Inputs=|+-
  Unit Delay : UnitDelay  SampleTime=-1  HasFrameUpgradeWarning=on
  derivative : Outport
  wires:
  e/1 -> Sum/1, Unit Delay/1
  Unit Delay/1 -> Sum/2
  Sum/1 -> Divide/1
  ATC input time constant/1 -> Data Type Conversion/1
  Divide/1 -> derivative/1
  Data Type Conversion/1 -> Divide/2

== system arducopter/Rate Controller/PID Roll Rate/I ==
  note: Integrator, see AC_PID::update_i()
  e : Inport
  limit_flg : Inport  Port=2
  ki : Inport  Port=3
  i_max : Inport  Port=4
  Constant1 : Constant  Value=sim.param.dt
  Data Type Conversion : DataTypeConversion  OutDataTypeStr=single
  IC1 : InitialCondition  Value=sim.init.PIDR.I
  Integrator : MATLAB Function  TreatAsAtomicUnit=on
  Unit Delay1 : UnitDelay  SampleTime=-1  HasFrameUpgradeWarning=on
  integrator : Outport
  wires:
  [integrator_out] -> integrator/1
  Constant1/1 -> Data Type Conversion/1
  limit_flg/1 -> Integrator/3(limit_flg)
  [integrator_out] -> Unit Delay1/1
  IC1/1 -> [integrator_out]
  Unit Delay1/1 -> Integrator/2(integrator)
  ki/1 -> Integrator/4(ki)
  i_max/1 -> Integrator/5(i_max)
  e/1 -> Integrator/1(error)
  Integrator/1(integrator_out) -> IC1/1
  Data Type Conversion/1 -> Integrator/6(dt)

== system arducopter/Rate Controller/PID Roll Rate/RAT_FLTD ==
  note: Digital Filter:
      | $y_n = (1 - \alpha)y_{n-1} + x \cdot \alpha$
  note: Alpha Calculation:
      | $\alpha = \frac{\mathrm{d}t}{\mathrm{d}t + 2 \pi T_{\mathrm{Cutoff}}$
  note: See AC_PID.cpp, update_all()
  note: See AP_Math.cpp, calc_lowpass_alpha_dt()
  u : Inport
  cutoff_freq : Inport  Port=2
  ATC input time constant : Constant  Value=sim.param.dt
  Add : Sum
  Calculate Alpha : Product  Inputs=*/
  Compare To Zero : simulink/Logic and Bit Operations/Compare To Zero  relop=<=  OutDataTypeStr=boolean
  Compare To Zero1 : simulink/Logic and Bit Operations/Compare To Zero  relop=<=  OutDataTypeStr=boolean
  Constant : Constant  Commented=on
  Constant1 : Constant  Commented=on
  Constant2 : Constant  OutDataTypeStr=single
  Constant3 : Constant  OutDataTypeStr=single
  Constant4 : Constant  OutDataTypeStr=single
  Data Type Conversion : DataTypeConversion  OutDataTypeStr=single
  Discrete Filter : DiscreteFilter  Commented=on  NumeratorSource=Input port  DenominatorSource=Input port  a0EqualsOne=on
  Divide : Product  Inputs=*/
  From : From  Commented=on  GotoTag=alpha
  From1 : From  Commented=on  GotoTag=alpha
  Gain : Gain  Gain=2*pi
  Gain1 : Gain  Commented=on  Gain=-1
  IC : InitialCondition  Value=sim.init.PIDR.DerFilt
  Logical Operator : Logic  Operator=OR  AllPortsSameDT=off  OutDataTypeStr=boolean
  Product : Product
  Product1 : Product
  Subtract : Sum  Commented=on  Inputs=+-
  Subtract1 : Sum  Inputs=+-
  Sum : Sum  Inputs=++|  AccumDataTypeStr=single
  Switch : Switch  Criteria=u2 > Threshold
  Unit Delay : UnitDelay  SampleTime=-1  HasFrameUpgradeWarning=on
  Vector Concatenate : Concatenate  Commented=on
  degree2radian1 : Gain  Commented=on  Gain=pi/180
  y : Outport
  wires:
  Product1/1 -> Sum/2
  Unit Delay/1 -> Product1/2
  Subtract1/1 -> Product1/1
  [alpha] -> Subtract1/2
  Constant2/1 -> Subtract1/1
  [alpha] -> Product/1
  Vector Concatenate/1 -> Discrete Filter/3
  Constant1/1 -> Vector Concatenate/1
  Gain1/1 -> Vector Concatenate/2
  Subtract/1 -> Gain1/1
  Constant/1 -> Subtract/1
  From1/1 -> Subtract/2
  From/1 -> Discrete Filter/2
  Calculate Alpha/1 -> Switch/3
  Add/1 -> Calculate Alpha/2
  [dt] -> Add/1, Calculate Alpha/1
  Gain/1 -> Divide/2
  cutoff_freq/1 -> [cutoff_freq]
  Discrete Filter/1 -> degree2radian1/1
  u/1 -> Product/2
  Divide/1 -> Add/2
  Constant3/1 -> Divide/1
  Product/1 -> Sum/1
  Switch/1 -> [alpha]
  ATC input time constant/1 -> Data Type Conversion/1
  [cutoff_freq] -> Gain/1
  [dt] -> Compare To Zero/1
  [cutoff_freq] -> Compare To Zero1/1
  Compare To Zero/1 -> Logical Operator/1
  Compare To Zero1/1 -> Logical Operator/2
  Logical Operator/1 -> Switch/2
  Constant4/1 -> Switch/1
  Sum/1 -> IC/1
  IC/1 -> Unit Delay/1, y/1
  Data Type Conversion/1 -> [dt]

== system arducopter/Rate Controller/PID Roll Rate/RAT_FLTE ==
  note: Digital Filter:
      | $y_n = (1 - \alpha)y_{n-1} + x \cdot \alpha$
  note: Alpha Calculation:
      | $\alpha = \frac{\mathrm{d}t}{\mathrm{d}t + 2 \pi f_{\mathrm{Cutoff}}$
  note: See AC_PID.cpp, update_all()
  note: See AP_Math.cpp, calc_lowpass_alpha_dt()
  u : Inport
  cutoff_freq : Inport  Port=2
  ATC input time constant : Constant  Value=sim.param.dt
  Add : Sum
  Calculate Alpha : Product  Inputs=*/
  Compare To Zero : simulink/Logic and Bit Operations/Compare To Zero  relop=<=  OutDataTypeStr=boolean
  Compare To Zero1 : simulink/Logic and Bit Operations/Compare To Zero  relop=<=  OutDataTypeStr=boolean
  Constant2 : Constant  OutDataTypeStr=single
  Constant3 : Constant  OutDataTypeStr=single
  Constant4 : Constant  OutDataTypeStr=single
  Data Type Conversion : DataTypeConversion  OutDataTypeStr=single
  Divide : Product  Inputs=*/
  Gain : Gain  Gain=2*pi
  IC : InitialCondition  Value=sim.init.PIDR.ErrFilt
  Logical Operator : Logic  Operator=OR  AllPortsSameDT=off  OutDataTypeStr=boolean
  Product : Product
  Product1 : Product
  Subtract1 : Sum  Inputs=+-
  Sum : Sum  Inputs=++|  OutDataTypeStr=single
  Switch : Switch  Criteria=u2 > Threshold
  Unit Delay : UnitDelay  SampleTime=-1  HasFrameUpgradeWarning=on
  y : Outport
  wires:
  Product1/1 -> Sum/2
  Unit Delay/1 -> Product1/2
  Subtract1/1 -> Product1/1
  [alpha] -> Subtract1/2
  Constant2/1 -> Subtract1/1
  [alpha] -> Product/1
  Calculate Alpha/1 -> Switch/3
  Add/1 -> Calculate Alpha/2
  [dt] -> Add/1, Calculate Alpha/1
  Gain/1 -> Divide/2
  cutoff_freq/1 -> [cutoff_freq]
  u/1 -> Product/2
  Divide/1 -> Add/2
  Constant3/1 -> Divide/1
  Product/1 -> Sum/1
  Switch/1 -> [alpha]
  ATC input time constant/1 -> Data Type Conversion/1
  [cutoff_freq] -> Gain/1
  [dt] -> Compare To Zero/1
  [cutoff_freq] -> Compare To Zero1/1
  Compare To Zero/1 -> Logical Operator/1
  Compare To Zero1/1 -> Logical Operator/2
  Logical Operator/1 -> Switch/2
  Constant4/1 -> Switch/1
  Sum/1 -> IC/1
  IC/1 -> Unit Delay/1, y/1
  Data Type Conversion/1 -> [dt]

== system arducopter/Rate Controller/PID Roll Rate/RAT_FLTT ==
  note: See AP_Math.cpp, calc_lowpass_alpha_dt()
  note: See AC_PID.cpp, update_all()
  note: Alpha Calculation:
      | $\alpha = \frac{\mathrm{d}t}{\mathrm{d}t + 2 \pi f_{\mathrm{Cutoff}}$
  note: Digital Filter:
      | $y_n = (1 - \alpha)y_{n-1} + x \cdot \alpha$
  u : Inport
  cutoff_freq : Inport  Port=2
  ATC input time constant : Constant  Value=sim.param.dt
  Add : Sum
  Calculate Alpha : Product  Inputs=*/
  Compare To Zero : simulink/Logic and Bit Operations/Compare To Zero  relop=<=  OutDataTypeStr=boolean
  Compare To Zero1 : simulink/Logic and Bit Operations/Compare To Zero  relop=<=  OutDataTypeStr=boolean
  Constant2 : Constant  OutDataTypeStr=single
  Constant3 : Constant  OutDataTypeStr=single
  Constant4 : Constant  OutDataTypeStr=single
  Data Type Conversion : DataTypeConversion  OutDataTypeStr=single
  Divide : Product  Inputs=*/
  Gain : Gain  Gain=2*pi
  IC : InitialCondition  Value=sim.init.PIDR.TarFilt
  Logical Operator : Logic  Operator=OR  AllPortsSameDT=off  OutDataTypeStr=boolean
  Product : Product
  Product1 : Product
  Subtract1 : Sum  Inputs=+-
  Sum : Sum  Inputs=++|
  Switch : Switch  Criteria=u2 > Threshold
  Unit Delay : UnitDelay  SampleTime=-1  HasFrameUpgradeWarning=on
  y : Outport
  wires:
  Constant4/1 -> Switch/1
  Logical Operator/1 -> Switch/2
  Compare To Zero1/1 -> Logical Operator/2
  Compare To Zero/1 -> Logical Operator/1
  [cutoff_freq] -> Compare To Zero1/1
  [dt] -> Compare To Zero/1
  [cutoff_freq] -> Gain/1
  ATC input time constant/1 -> Data Type Conversion/1
  Switch/1 -> [alpha]
  Product/1 -> Sum/1
  Constant3/1 -> Divide/1
  Divide/1 -> Add/2
  u/1 -> Product/2
  cutoff_freq/1 -> [cutoff_freq]
  Gain/1 -> Divide/2
  [dt] -> Calculate Alpha/1, Add/1
  Add/1 -> Calculate Alpha/2
  Calculate Alpha/1 -> Switch/3
  [alpha] -> Product/1
  Constant2/1 -> Subtract1/1
  [alpha] -> Subtract1/2
  Subtract1/1 -> Product1/1
  Product1/1 -> Sum/2
  Sum/1 -> IC/1
  Unit Delay/1 -> Product1/2
  IC/1 -> y/1, Unit Delay/1
  Data Type Conversion/1 -> [dt]
